simulink model "LM35_TEMP"  (R2018b)
settings: Solver=FixedStepAuto  StartTime=0.0  StopTime=inf  RelTol=1e-3  EnableMultiTasking=on
settings Model: ExtModeTrigDuration=2  Creator=munir  LastModifiedBy=munir
settings OptimizationCC: EnhancedBackFolding=on  PassReuseOutputArgsAs=Individual arguments  MaxStackSize=64  OptimizeBlockOrder=speed  DifferentSizesBufferReuse=on  OptimizationCustomize=off
settings DebuggingCC: ParameterTunabilityLossMsg=error
settings HardwareCC: ProdBitPerInt=16  ProdBitPerPointer=16  ProdBitPerSizeT=16  ProdBitPerPtrDiffT=16  ProdLargestAtomicFloat=None  ProdWordSize=8  ProdHWDeviceType=Atmel->AVR
settings SFSimCC: MATLABDynamicMemAlloc=off
settings RTWCC: SystemTargetFile=ert.tlc  HardwareBoard=Arduino Mega 2560  TemplateMakefile=ert_default_tmf  GenerateReport=on  Toolchain=Arduino AVR  BuildConfiguration=Faster Runs  IncludeHyperlinkInReport=on  LaunchReport=on  GenerateTraceInfo=on  GenerateTraceReport=on  GenerateTraceReportSl=on  GenerateTraceReportSf=on  GenerateTraceReportEml=on
settings CodeAppCC: ForceParamTrailComments=on  IgnoreCustomStorageClasses=off  OperatorAnnotations=on  SimulinkDataObjDesc=on  SFDataObjDesc=on  InsertBlockDesc=on
settings ERTTargetCC: SupportContinuousTime=on  SupportVariableSizeSignals=on

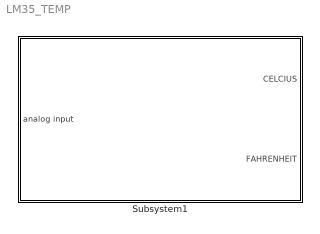
== system LM35_TEMP ==
  Subsystem1 : Subsystem

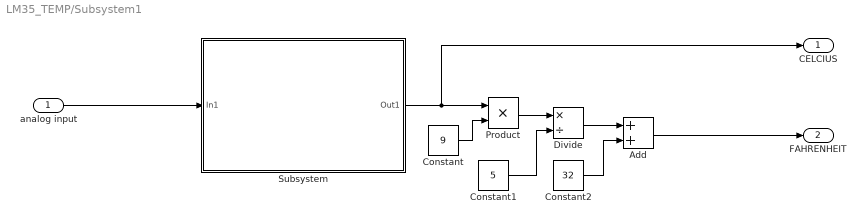
== system LM35_TEMP/Subsystem1 ==
  analog input : Inport
  Add : Sum
  Constant : Constant  Value=9
  Constant1 : Constant  Value=5
  Constant2 : Constant  Value=32
  Divide : Product  Inputs=*/
  Product : Product
  Subsystem : Subsystem
  CELCIUS : Outport
  FAHRENHEIT : Outport  Port=2
  wires:
  Constant/1 -> Product/2
  Divide/1 -> Add/1
  Product/1 -> Divide/1
  Subsystem/1(Out1) -> CELCIUS/1, Product/1
  analog input/1 -> Subsystem/1(In1)
  Constant2/1 -> Add/2
  Constant1/1 -> Divide/2
  Add/1 -> FAHRENHEIT/1

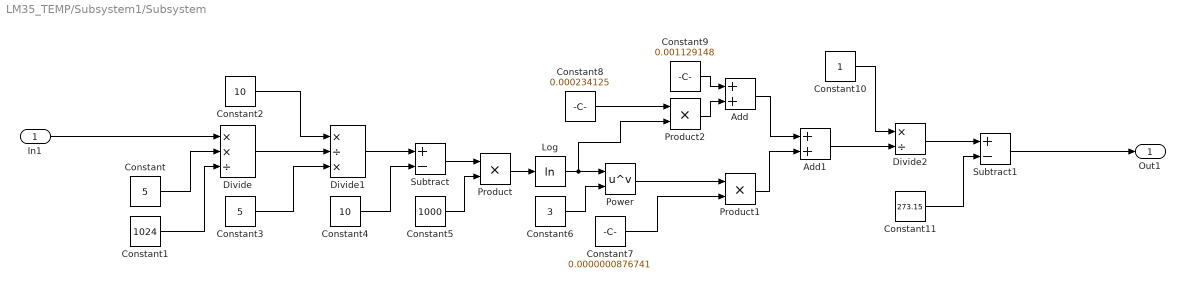
== system LM35_TEMP/Subsystem1/Subsystem ==
  In1 : Inport
  Add : Sum
  Add1 : Sum
  Constant : Constant  Value=5
  Constant1 : Constant  Value=1024
  Constant10 : Constant
  Constant11 : Constant  Value=273.15
  Constant2 : Constant  Value=10
  Constant3 : Constant  Value=5
  Constant4 : Constant  Value=10
  Constant5 : Constant  Value=1000
  Constant6 : Constant  Value=3
  Constant7 : Constant  Value=0.0000000876741
  Constant8 : Constant  Value=0.000234125
  Constant9 : Constant  Value=0.001129148
  Divide : Product  Inputs=**/
  Divide1 : Product  Inputs=*/*
  Divide2 : Product  Inputs=*/
  Log : Math  Operator=log  SaturateOnIntegerOverflow=on
  Power : Math  Operator=pow  SaturateOnIntegerOverflow=on
  Product : Product
  Product1 : Product
  Product2 : Product
  Subtract : Sum  Inputs=+-
  Subtract1 : Sum  Inputs=+-
  Out1 : Outport
  wires:
  Subtract1/1 -> Out1/1
  Log/1 -> Product2/2, Power/1
  Constant2/1 -> Divide1/1
  Subtract/1 -> Product/1
  Constant11/1 -> Subtract1/2
  Constant8/1 -> Product2/1
  Constant/1 -> Divide/2
  Divide/1 -> Divide1/2
  Add1/1 -> Divide2/2
  Product2/1 -> Add/2
  Constant10/1 -> Divide2/1
  Constant1/1 -> Divide/3
  Product/1 -> Log/1
  Constant4/1 -> Subtract/2
  Constant6/1 -> Power/2
  Constant9/1 -> Add/1
  Divide2/1 -> Subtract1/1
  Add/1 -> Add1/1
  Product1/1 -> Add1/2
  Constant3/1 -> Divide1/3
  Constant5/1 -> Product/2
  Power/1 -> Product1/1
  Divide1/1 -> Subtract/1
  Constant7/1 -> Product1/2
  In1/1 -> Divide/1
